simulink model "Ebike_FaultModel_2"  (R2024b)
settings: Solver=VariableStepAuto  StartTime=0.0  StopTime=20.0  RelTol=1e-3  EnableMultiTasking=on
settings Model: Creator=s.maatoug  LastModifiedBy=s.maatoug
settings DebuggingCC: InheritedTsInSrcMsg=none

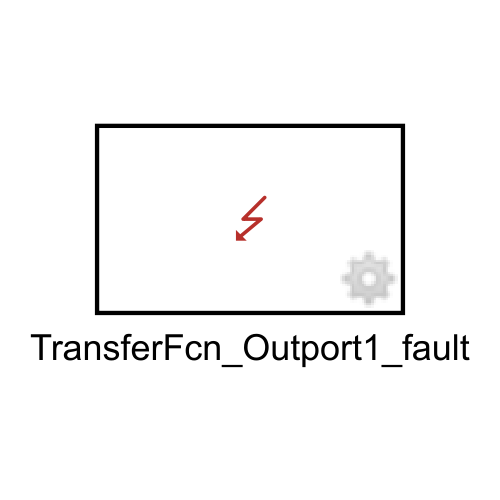
[thumbnail: Simulink's stored preview of the top-level diagram]
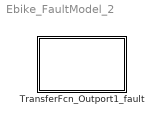
== system Ebike_FaultModel_2 ==
  TransferFcn_Outport1_fault : Subsystem  TreatAsAtomicUnit=on  IsInjectorSS=on

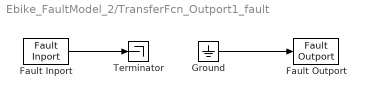
== system Ebike_FaultModel_2/TransferFcn_Outport1_fault ==
  Fault Inport : FaultInport
  Fault Outport : FaultOutport
  Ground : Ground
  Terminator : Terminator
  wires:
  Ground/1 -> Fault Outport/1
  Fault Inport/1 -> Terminator/1
